simulink model "SFR_WG"  (R2022b)
settings: Solver=VariableStepAuto  StartTime=0.0  StopTime=tsimulation  RelTol=1e-3
values from neighbouring files (symbols this model uses):
  Hw = 5    [WGmodel_startup.m]    (also in WGmodel_startup_v2.m; WGmodel_startup_v3.m)
  m_pw = zeros(nvw,nwr)    [fun_getwindpowercurve_v4.m]
  pinitwindgen = 0.5161    [WGmodel_startup.m]    (also in WGmodel_startup_v2.m; WGmodel_startup_v3.m = pinitwindgen(1))
  R = 0.05    [WGmodel_startup.m]    (also in WGmodel_startup_v2.m; WGmodel_startup_v3.m)
  Tc1 = 0.05    [WGmodel_startup.m]    (also in WGmodel_startup_v2.m; WGmodel_startup_v3.m)
  Tc2 = 0.05    [WGmodel_startup.m]    (also in WGmodel_startup_v2.m; WGmodel_startup_v3.m)
  v_pwdel = 0.9 * max(m_pw,[],2)    [fun_getwindpowercurve_v2.m]    (also in fun_getwindpowercurve_v3.m = (1-deload) * v_pwmpp; fun_getwindpowercurve_v4.m = (1-deload) * v_pwmpp)
  v_vw = 5:10    [LUT_2D.m]    (also in WGmodel_startup.m = 5:1:10; WGmodel_startup_v2.m = 5:1:15; WGmodel_startup_v3.m = 5:.5:12; fun_getwindpowercurve_v2.m = [10 11 12])
  v_wr = v_Wr/Wrn    [fun_getwindpowercurve.m]    (also in fun_getwindpowercurve_v2.m; fun_getwindpowercurve_v3.m; fun_getwindpowercurve_v4.m; fun_getwindpowercurve_v5.m)
  v_wrdel = (v_wr(v_iwrmpp+i_lower)+v_wr(v_iwrmpp+i_higher))/2    [fun_getwindpowercurve_v2.m]    (also in fun_getwindpowercurve_v3.m = v_Wrdel/Wrn; fun_getwindpowercurve_v4.m = v_Wrdel/Wrn)
  wr0 = wr0(1)    [WGmodel_startup_v3.m]
settings Model: Creator=lsigrist  LastModifiedBy=User
settings SolverCC: AlgebraicLoopSolver=TrustRegion
settings DataIOCC: FinalStateName=xInitial  LoadInitialState=on  SaveOutput=off  SignalLogging=off  DSMLogging=off  ReturnWorkspaceOutputs=off
settings DebuggingCC: UnconnectedInputMsg=warning  UnconnectedOutputMsg=warning  UnconnectedLineMsg=warning  SFMachineParentedDataDiag=warning  ArithmeticOperatorsInVariantConditions=warning
settings ModelReferenceCC: EnableRefExpFcnMdlSchedulingChecks=on
settings SFSimCC: CustomCodeUndefinedFunction=UseInterfaceOnly
settings RTWCC: DLArmComputeVersion=19.05

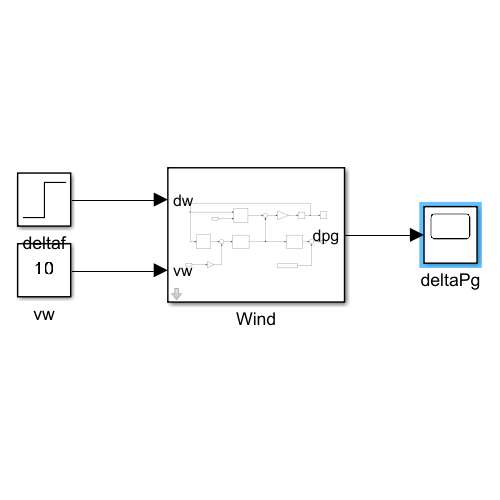
[thumbnail: Simulink's stored preview of the top-level diagram]
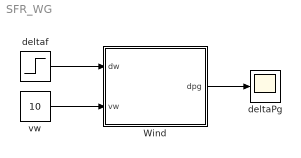
== system SFR_WG ==
  Wind : Subsystem  mask{Hw=Hw, Tc1=Tc1, Tc2=Tc2, pinitwindgen=pinitwindgen, wr0=wr0, v_vw=v_vw, v_wr=v_wr, m_pw=m_pw, v_wrdel=v_wrdel, v_pwdel=v_pwdel}
      mask prompts: Hw "Rotor inertia (s)"; Tc1 "MSC time constant (s)"; Tc2 "GSC time constant (s)"; pinitwindgen "Initial power (pu)"; wr0 "Initial rotor speed (pu)"; v_vw "Wind speed (m/s)"; v_wr "Rotor speed (pu)"; m_pw "Mechanical power (pu)"; v_wrdel "Deloaded rotor speed (pu)"; v_pwdel "Deloaded electrical power (pu)"
      mask DialogControl Container5 Prompt: Operation point
      mask DialogControl Container5_copy Prompt: Power-speed curves
  deltaPg : Scope
  deltaf : Step  Time=100  After=0.05  SampleTime=0
  vw : Constant  Value=10
  wires:
  vw/1 -> Wind/2(vw)
  Wind/1(dpg) -> deltaPg/1
  deltaf/1 -> Wind/1(dw)

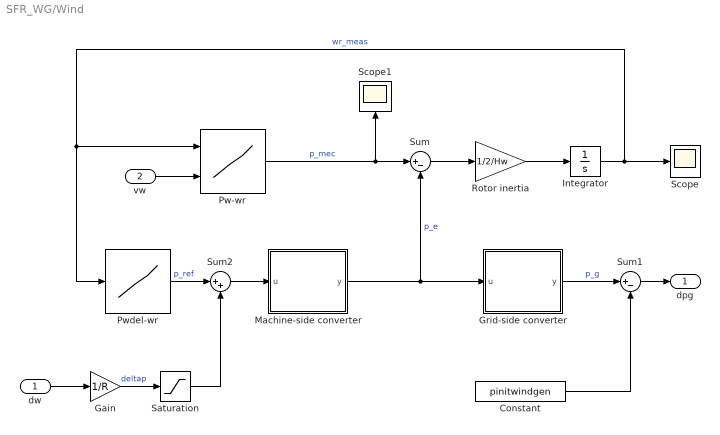
== system SFR_WG/Wind ==
  dw : Inport
  vw : Inport  Port=2
  Constant : Constant  Value=pinitwindgen
  Gain : Gain  Gain=1/R
  Grid-side converter : Subsystem  mask{T=Tc2, y0=pinitwindgen}
      mask prompts: T "Time constant (s)"; y0 "Initial condition (pu)"
  Integrator : Integrator  InitialCondition=wr0
  Machine-side converter : Subsystem  mask{T=Tc1, y0=pinitwindgen}
      mask prompts: T "Time constant (s)"; y0 "Initial condition (pu)"
  Pw-wr : Lookup_n-D  BreakpointsForDimension1=v_vw  BreakpointsForDimension2=v_wr  Table=m_pw  InternalRulePriority=Speed  RndMeth=Simplest
      settings: InputPortMap=u0,u1
  Pwdel-wr : Lookup_n-D  NumberOfTableDimensions=1  BreakpointsForDimension1=v_wrdel  Table=v_pwdel  InternalRulePriority=Speed  RndMeth=Simplest
  Rotor inertia : Gain  Gain=1/2/Hw
  Saturation : Saturate  UpperLimit=v_pwdel(length(v_pwdel))  LowerLimit=0
  Scope : Scope
  Scope1 : Scope
  Sum : Sum  Inputs=|+-
  Sum1 : Sum  Inputs=|+-
  Sum2 : Sum  Inputs=|++
  dpg : Outport  VectorParamsAs1DForOutWhenUnconnected=off
  wires:
  Pw-wr/1 -> Scope1/1, Sum/1  "p_mec"
  Sum/1 -> Rotor inertia/1
  Machine-side converter/1(y) -> Grid-side converter/1(u), Sum/2  "p_e"
  Integrator/1 -> Pwdel-wr/1, Pw-wr/1, Scope/1  "wr_meas"
  Rotor inertia/1 -> Integrator/1
  dw/1 -> Gain/1
  vw/1 -> Pw-wr/2
  Grid-side converter/1(y) -> Sum1/1  "p_g"
  Sum1/1 -> dpg/1
  Constant/1 -> Sum1/2
  Gain/1 -> Saturation/1  "deltap"
  Pwdel-wr/1 -> Sum2/1  "p_ref"
  Sum2/1 -> Machine-side converter/1(u)
  Saturation/1 -> Sum2/2

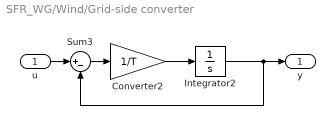
== system SFR_WG/Wind/Grid-side converter ==
  u : Inport
  Converter2 : Gain  Gain=1/T
  Integrator2 : Integrator  InitialCondition=y0
  Sum3 : Sum  Inputs=|+-
  y : Outport
  wires:
  Integrator2/1 -> y/1, Sum3/2
  Sum3/1 -> Converter2/1
  Converter2/1 -> Integrator2/1
  u/1 -> Sum3/1

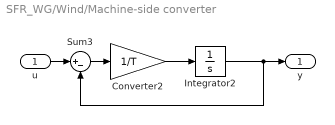
== system SFR_WG/Wind/Machine-side converter ==
  u : Inport
  Converter2 : Gain  Gain=1/T
  Integrator2 : Integrator  InitialCondition=y0
  Sum3 : Sum  Inputs=|+-
  y : Outport
  wires:
  Integrator2/1 -> y/1, Sum3/2
  Sum3/1 -> Converter2/1
  Converter2/1 -> Integrator2/1
  u/1 -> Sum3/1
